simulink model "Cell_model_final4"  (R2023a)
settings: Solver=VariableStepAuto  StartTime=0.0  StopTime=T_e  FixedStep=0.005  RelTol=0.1
undefined symbols (not defined in the file or in its folder): C1_253, C1_263, C1_273, C1_283, C1_298, OCV_253, OCV_263, OCV_273, OCV_283, OCV_298, R0_253, R0_263, R0_273, R0_283, R0_298, R1_253, R1_263, R1_273, R1_283, R1_298
libraries: nesl_utility x8, fl_lib x7, dspstat3 x3, BatteryEstimators x1, deeplib x1, ee_lib x1, spspowerguiLib x1
settings Model: Creator=Lenovo  LastModifiedBy=Lenovo
settings DebuggingCC: AlgebraicLoopMsg=none

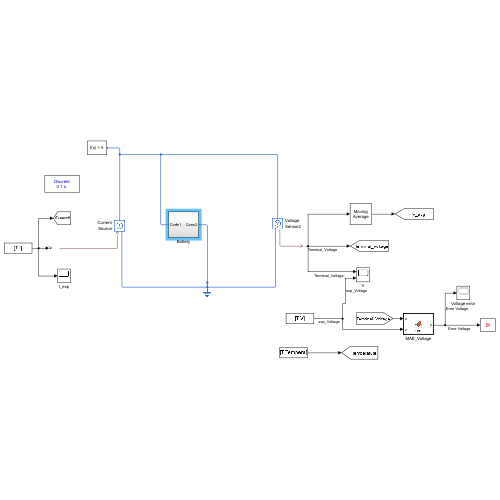
[thumbnail: Simulink's stored preview of the top-level diagram]
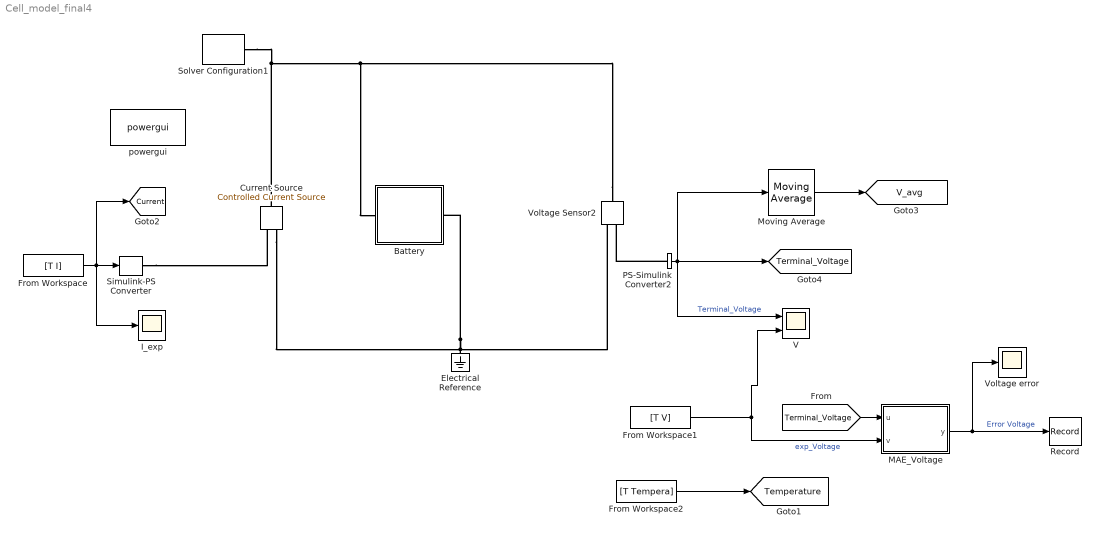
== system Cell_model_final4 ==
  Battery : Subsystem
  Current Source : fl_lib/Electrical/Electrical Sources/Controlled Current Source
  Electrical Reference : fl_lib/Electrical/Electrical Elements/Electrical Reference
  From Workspace : FromWorkspace  VariableName=[T I]
  From Workspace1 : FromWorkspace  VariableName=[T V]
  From Workspace2 : FromWorkspace  VariableName=[T Tempera]
  I_exp : Scope
  MAE_Voltage : MATLAB Function  TreatAsAtomicUnit=on
  Moving Average : dspstat3/Moving Average  Method=Sliding window  ForgettingFactorPort=off  SpecifyWindowLength=on  WindowLength=600  OverlapLength=599  AllowArbitraryInputLength=off  ForgettingFactor=0.9  SimulateUsing=Code generation
  PS-Simulink Converter2 : nesl_utility/PS-Simulink Converter  PhysicalDomain=network_engine_domain  SubClassName=ps_output  LeftPortType=input  RightPortType=output  PseudoPeriodic=off  Frequencies=[]  VectorFormat=1-D array  Unit=V  AffineConversion=off
  Record : Record  FileSettingsInternal="{\"entries\":[{\"content\":{\"excelSettings\":{\"content\":{},\"type\":\"Streamout.ExcelSettings\"}},\"type\":\"Streamout.FileSettingStorage\",\"uuid\":\"ccaf1daf-0eb7-4141-93b9-257bac153734\"}],\"packageUris\":[\"http://schema.mathworks.com/mf0/streamout_blocks/R2020a\"],\"version\":\"1.0\"}"  SignalsInternal="{\"entries\":[{\"content\":{\"signals\":[{\"content\":{\"blockPath\":[\"Cell_model_final4/Record\"],\"dimensions\":[1],\"domain\":\"Cell_model_final4/Record\",\"lineColor\":\"#a2142f\",\"plots\":[1],\"port\":1,\"sid\":[\"\"],\"signalID\":228,\"signalName\":\"Error Voltage\"},\"type\":\"RecordBlkView.Signal\",\"uuid\":\"8161d02f-5d6f-4f2d-b72f-e0f8d4715f56\"}]},\"type\":\"RecordBlkView.InputSignals\",\"uuid\":\"ac346876-ca78-426d-94f9-f8beec700152\"}],\"packageUris\":[\"http://schema.mathworks.com/mf0/streamout_blocks/R2020a\"],\"version\":\"1.0\"}"  VisualizationBindings="{\"sparklinesplugin\":{\"info\":[{\"bindingParametersList\":[],\"subplotID\":1}]}}"
  Simulink-PS Converter : nesl_utility/Simulink-PS Converter  PhysicalDomain=network_engine_domain  SubClassName=ps_input  LeftPortType=input  RightPortType=output  PseudoPeriodic=off  Frequencies=[]  NoiseDistribution=none  NoiseParameters=[]  Unit=A  AffineConversion=off  FilteringAndDerivatives=zero  SimscapeFilterOrder=1  InputFilterTimeConstant=.001  UdotUserProvided=0
  Solver Configuration1 : nesl_utility/Solver Configuration  PhysicalDomain=network_engine_domain  SubClassName=solver  LeftPortType=input  RightPortType=generic  Tones=[]  Harmonics=[]  SimulateNoise=off  Profile=off  UseLocalSampling=off  EnableSwitchedLinearOptims=on  FrequencyDomain=off  UseCCode=off  RelTol=0.001  AbsTol=0.001  MinStep=1e-09  ToWorkspace=off  RevertToSquareIcSolve=off  NumHomotopyIterations=100  PhasorMode=off  PhasorModeNumHarmonics=1  ConsistencySolver=NEWTON_XTOL_AFTER_FTOL  IndexReductionMethod=DerivativeReplacement  DoDC=off  ResidualTolerance=1e-09  ConsistencyTolSource=GLOBAL  ConsistencyAbsTol=0.001  ConsistencyRelTol=0.001  ConsistencyTolFactor=0.001  UseLocalSolver=off  LocalSolverChoice=NE_BACKWARD_EULER_ADVANCER  ResolveIndetEquations=on  FunctionEvalNumThread=1  LocalSolverSampleTime=0.001  DoFixedCost=off  MaxNonlinIter=3  MaxModeIter=2  ComputeImpulses=off  ImpulseIterations=2  LinearAlgebra=auto  LinearAlgebraNumThread=0  EquationFormulation=NE_TIME_EF  DelaysMemoryBudget=1024  AutomaticFiltering=on  FilteringTimeConstant=0.001  PartitionStorageMethod=AS_NEEDED  PartitionMemoryBudget=1024  PartitionMethod=ROBUST
  V : Scope  NumInputPorts=2
  Voltage Sensor2 : fl_lib/Electrical/Electrical Sensors/Voltage Sensor
  Voltage error : Scope
  powergui : spspowerguiLib/powergui  Priority=1  SimulationMode=Discrete  SampleTime=0.1  frequency=60  Iterations=50  frequencyindice=60  Pbase=100e6  ErrMax=1e-4  UnitsV=kV  UnitsW=MW  buscounter=0  FunctionMessages=off  echomessages=off  EnableUseOfTLC=off  CurrentSourceSwitches=off  DisableSnubberDevices=off  DisableRonSwitches=off  DisableVfSwitches=off  DisplayEquations=off  AutomaticDiscreteSolvers=off  SolverType=Tustin/Backward Euler (TBE)  Interpol=off  ExternalGateDelay=off  methode=off  Ts=100  x0status=blocks  SPID=on  SwTol=0  HookPort=off  NonlinearTolerance=1e-4  nMaxIteration=100  ContinueOnMaxIteration=off  RestoreLinks=warning  ResistiveCurrentMeasurement=off  Frange=[0:2:500]  Ylog=off  Xlog=on  ShowGrid=off  save=off  variable=ZData  structure=0  ZoomFFT=off  StartTime=0.0  cycles=1  DisplayStyle=1  fundamental=60  FreqAxis=off  MaxFrequency=1000  frequencyindicesteady=1  RmsSteady=1  display=off
  tag scope: Current=global, Temperature=global, Terminal_Voltage=global, V_avg=global
  wires:
  Moving Average/1 -> [V_avg]
  PS-Simulink Converter2/1 -> Moving Average/1, V/1, [Terminal_Voltage]  "Terminal_Voltage"
  From Workspace/1 -> I_exp/1, [Current], Simulink-PS Converter/1
  MAE_Voltage/1(y) -> Voltage error/1, Record/1  "Error Voltage"
  From Workspace1/1 -> V/2, MAE_Voltage/2(v)  "exp_Voltage"
  From Workspace2/1 -> [Temperature]
  [Terminal_Voltage] -> MAE_Voltage/1(u)
  connections:
  Voltage Sensor2/RConn2 -- Current Source/RConn2 -- Electrical Reference/LConn1 -- Battery/RConn1
  Voltage Sensor2/LConn1 -- Solver Configuration1/RConn1 -- Current Source/LConn1 -- Battery/LConn1
  Simulink-PS Converter/RConn1 -- Current Source/RConn1
  PS-Simulink Converter2/LConn1 -- Voltage Sensor2/RConn1

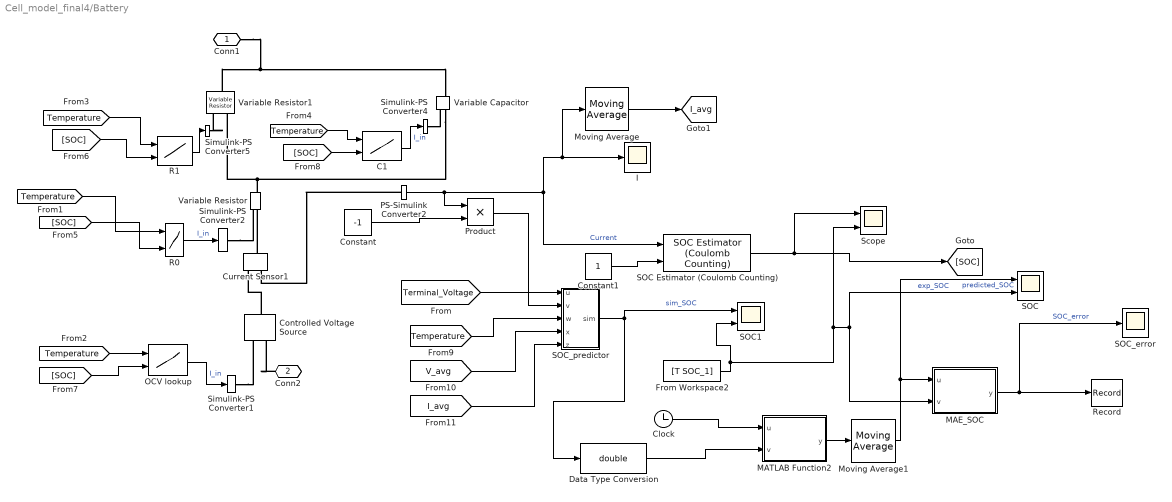
== system Cell_model_final4/Battery ==
  C1 : Lookup_n-D  BreakpointsForDimension1=[253;263;273;283;298]  BreakpointsForDimension2=[0;0.1;0.2;0.3;0.4;0.5;0.6;0.7;0.8;0.9;1]  Table=[C1_253;C1_263;C1_273;C1_283;C1_298]  InternalRulePriority=Speed  RndMeth=Simplest
      settings: InputPortMap=u0,u1
  Clock : Clock
  Constant : Constant  Value=-1
  Constant1 : Constant
  Controlled Voltage Source : fl_lib/Electrical/Electrical Sources/Controlled Voltage Source
  Current Sensor1 : fl_lib/Electrical/Electrical Sensors/Current Sensor
  Data Type Conversion : DataTypeConversion  OutDataTypeStr=double  SaturateOnIntegerOverflow=off  RndMeth=Floor
  From Workspace2 : FromWorkspace  VariableName=[T SOC_1]
  I : Scope
  MAE_SOC : MATLAB Function  TreatAsAtomicUnit=on
  MATLAB Function2 : MATLAB Function  TreatAsAtomicUnit=on
  Moving Average : dspstat3/Moving Average  Method=Sliding window  ForgettingFactorPort=off  SpecifyWindowLength=on  WindowLength=600  OverlapLength=599  AllowArbitraryInputLength=off  ForgettingFactor=0.9  SimulateUsing=Code generation
  Moving Average1 : dspstat3/Moving Average  Method=Sliding window  ForgettingFactorPort=off  SpecifyWindowLength=on  WindowLength=600  OverlapLength=599  AllowArbitraryInputLength=off  ForgettingFactor=0.9  SimulateUsing=Code generation
  OCV lookup : Lookup_n-D  BreakpointsForDimension1=[253;263;273;283;298]  BreakpointsForDimension2=[0;0.1;0.2;0.3;0.4;0.5;0.6;0.7;0.8;0.9;1]  Table=[OCV_253;OCV_263;OCV_273;OCV_283;OCV_298]  InternalRulePriority=Speed  RndMeth=Simplest
      settings: InputPortMap=u0,u1
  PS-Simulink Converter2 : nesl_utility/PS-Simulink Converter  PhysicalDomain=network_engine_domain  SubClassName=ps_output  LeftPortType=input  RightPortType=output  PseudoPeriodic=off  Frequencies=[]  VectorFormat=1-D array  Unit=A  AffineConversion=off
  Product : Product
  R0 : Lookup_n-D  BreakpointsForDimension1=[253;263;273;283;298]  BreakpointsForDimension2=[0;0.1;0.2;0.3;0.4;0.5;0.6;0.7;0.8;0.9;1]  Table=[R0_253;R0_263;R0_273;R0_283;R0_298]  InternalRulePriority=Speed  RndMeth=Simplest
      settings: InputPortMap=u0,u1
  R1 : Lookup_n-D  BreakpointsForDimension1=[253;263;273;283;298]  BreakpointsForDimension2=[0;0.1;0.2;0.3;0.4;0.5;0.6;0.7;0.8;0.9;1]  Table=[R1_253;R1_263;R1_273;R1_283;R1_298]  InternalRulePriority=Speed  RndMeth=Simplest
      settings: InputPortMap=u0,u1
  Record : Record  FileSettingsInternal="{\"entries\":[{\"content\":{\"excelSettings\":{\"content\":{},\"type\":\"Streamout.ExcelSettings\"}},\"type\":\"Streamout.FileSettingStorage\",\"uuid\":\"4492bafd-2dc4-4cd0-8cf0-f61798b460af\"}],\"packageUris\":[\"http://schema.mathworks.com/mf0/streamout_blocks/R2020a\"],\"version\":\"1.0\"}"  SignalsInternal="{\"entries\":[{\"content\":{\"signals\":[{\"content\":{\"blockPath\":[\"Cell_model_final4/Battery/Record\"],\"dimensions\":[1],\"domain\":\"Cell_model_final4/Battery/Record\",\"lineColor\":\"#139fff\",\"plots\":[1],\"port\":1,\"sid\":[\"\"],\"signalID\":232,\"signalName\":\"SOC_error\"},\"type\":\"RecordBlkView.Signal\",\"uuid\":\"cd1a7c72-596a-4650-bde3-9b31eae5e432\"}]},\"type\":\"RecordBlkView.InputSignals\",\"uuid\":\"78da0c69-a6e8-451d-b8ce-dbeaf7244afc\"}],\"packageUris\":[\"http://schema.mathworks.com/mf0/streamout_blocks/R2020a\"],\"version\":\"1.0\"}"  VisualizationBindings="{\"sparklinesplugin\":{\"info\":[{\"bindingParametersList\":[],\"subplotID\":1}]}}"
  SOC : Scope  NumInputPorts=2
  SOC Estimator (Coulomb Counting) : BatteryEstimators/SOC Estimator (Coulomb Counting)  AH=2.9  Ts=1
      settings: LibrarySourceBlock=|
      | batt_sl_lib/Estimators/SOC Estimator
      | (Coulomb Counting)
  SOC1 : Scope  NumInputPorts=2
  SOC_error : Scope
  SOC_predictor : Subsystem
  Scope : Scope  NumInputPorts=2
  Simulink-PS Converter1 : nesl_utility/Simulink-PS Converter  PhysicalDomain=network_engine_domain  SubClassName=ps_input  LeftPortType=input  RightPortType=output  PseudoPeriodic=off  Frequencies=[]  NoiseDistribution=none  NoiseParameters=[]  Unit=V  AffineConversion=off  FilteringAndDerivatives=zero  SimscapeFilterOrder=1  InputFilterTimeConstant=.001  UdotUserProvided=0
  Simulink-PS Converter2 : nesl_utility/Simulink-PS Converter  PhysicalDomain=network_engine_domain  SubClassName=ps_input  LeftPortType=input  RightPortType=output  PseudoPeriodic=off  Frequencies=[]  NoiseDistribution=none  NoiseParameters=[]  Unit=Ohm  AffineConversion=off  FilteringAndDerivatives=zero  SimscapeFilterOrder=1  InputFilterTimeConstant=.001  UdotUserProvided=0
  Simulink-PS Converter4 : nesl_utility/Simulink-PS Converter  PhysicalDomain=network_engine_domain  SubClassName=ps_input  LeftPortType=input  RightPortType=output  PseudoPeriodic=off  Frequencies=[]  NoiseDistribution=none  NoiseParameters=[]  Unit=F  AffineConversion=off  FilteringAndDerivatives=zero  SimscapeFilterOrder=1  InputFilterTimeConstant=.001  UdotUserProvided=0
  Simulink-PS Converter5 : nesl_utility/Simulink-PS Converter  PhysicalDomain=network_engine_domain  SubClassName=ps_input  LeftPortType=input  RightPortType=output  PseudoPeriodic=off  Frequencies=[]  NoiseDistribution=none  NoiseParameters=[]  Unit=Ohm  AffineConversion=on  FilteringAndDerivatives=provide  SimscapeFilterOrder=1  InputFilterTimeConstant=0.001  UdotUserProvided=0
  Variable Capacitor : ee_lib/Passive/Variable Capacitor  prm=2  Cmin=1e-9 F  r=1e-6 Ohm  v0=0 V  q0=0 C
      settings: InternalSimscapePortConfiguration="{\"Bottom\":[],\"Left\":[{\"id\":\"C\",\"label\":\"C\",\"type\":\"input\"},{\"id\":\"p\",\"label\":\"+\",\"type\":\"foundation.electrical.electrical\"}],\"Right\":[{\"id\":\"n\",\"label\":\"-\",\"type\":\"foundation.electrical.electrical\"}],\"Top\":[]}"
  Variable Resistor : fl_lib/Electrical/Electrical Elements/Variable Resistor  Rmin=0 Ohm  i_specify=off  i_priority=None  i=0 A  i_nominal_specify=off  i_nominal_unit=A  i_nominal_value=1  v_specify=off  v_priority=None  v=0 V  v_nominal_specify=off  v_nominal_unit=V  v_nominal_value=1
  Variable Resistor1 : fl_lib/Electrical/Electrical Elements/Variable Resistor  Rmin=0 Ohm  i_specify=off  i_priority=None  i=0 A  i_nominal_specify=off  i_nominal_unit=A  i_nominal_value=1  v_specify=off  v_priority=None  v=0 V  v_nominal_specify=off  v_nominal_unit=V  v_nominal_value=1
  Conn1 : PMIOPort  Side=Left
  Conn2 : PMIOPort  Port=2  Side=Right
  tag scope: I_avg=global
  wires:
  [Temperature] -> R0/1
  [SOC] -> R0/2
  [SOC] -> R1/2
  [Temperature] -> R1/1
  R1/1 -> Simulink-PS Converter5/1
  C1/1 -> Simulink-PS Converter4/1  "I_in"
  [Temperature] -> C1/1
  [SOC] -> C1/2
  PS-Simulink Converter2/1 -> Moving Average/1, I/1, SOC Estimator (Coulomb Counting)/1, Product/1  "Current"
  [Temperature] -> SOC_predictor/3(w)
  From Workspace2/1 -> SOC1/2, Scope/2, MAE_SOC/2(v), SOC/2  "exp_SOC"
  [Terminal_Voltage] -> SOC_predictor/1(u)
  [SOC] -> OCV lookup/2
  [Temperature] -> OCV lookup/1
  OCV lookup/1 -> Simulink-PS Converter1/1  "I_in"
  R0/1 -> Simulink-PS Converter2/1  "I_in"
  MAE_SOC/1(y) -> SOC_error/1, Record/1  "SOC_error"
  [V_avg] -> SOC_predictor/4(x)
  Moving Average/1 -> [I_avg]
  [I_avg] -> SOC_predictor/5(z)
  Constant/1 -> Product/2
  Product/1 -> SOC_predictor/2(v)
  Clock/1 -> MATLAB Function2/1(u)
  SOC_predictor/1(sim) -> SOC1/1, Data Type Conversion/1  "sim_SOC"
  Data Type Conversion/1 -> MATLAB Function2/2(v)
  SOC Estimator (Coulomb Counting)/1 -> Scope/1, [SOC]
  MATLAB Function2/1(y) -> Moving Average1/1
  Constant1/1 -> SOC Estimator (Coulomb Counting)/2
  Moving Average1/1 -> MAE_SOC/1(u), SOC/1  "predicted_SOC"
  connections:
  Simulink-PS Converter4/RConn1 -- Variable Capacitor/LConn1
  Simulink-PS Converter5/RConn1 -- Variable Resistor1/LConn1
  Variable Resistor/RConn1 -- Variable Resistor1/LConn2 -- Variable Capacitor/LConn2
  Simulink-PS Converter1/RConn1 -- Controlled Voltage Source/RConn1
  Variable Resistor1/RConn1 -- Conn1/RConn1 -- Variable Capacitor/RConn1
  Conn2/RConn1 -- Controlled Voltage Source/RConn2
  Simulink-PS Converter2/RConn1 -- Variable Resistor/LConn1
  Controlled Voltage Source/LConn1 -- Current Sensor1/RConn2
  Current Sensor1/LConn1 -- Variable Resistor/LConn2
  PS-Simulink Converter2/LConn1 -- Current Sensor1/RConn1

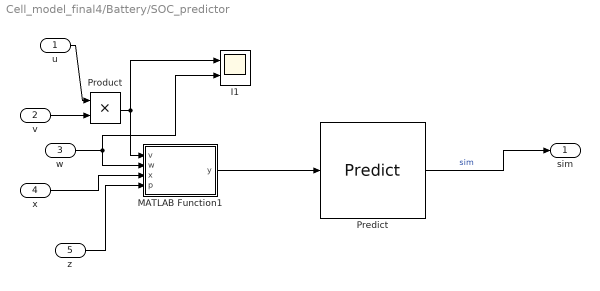
== system Cell_model_final4/Battery/SOC_predictor ==
  u : Inport
  v : Inport  Port=2
  w : Inport  Port=3
  x : Inport  Port=4
  z : Inport  Port=5
  I1 : Scope  NumInputPorts=2
  MATLAB Function1 : MATLAB Function  TreatAsAtomicUnit=on
  Predict : deeplib/Predict  Network=Network from MAT-file  NetworkFunction=squeezenet  NetworkFilePath=D:\Projects\Final_Year_Project\simulation\our_simulation\nets9.mat  MiniBatchSize=1  InputDataFormats={'',''}  Predictions=on  Activations={}  ForceInterpretedSim=off  EnableDLNetwork=on
  Product : Product
  sim : Outport
  wires:
  u/1 -> Product/1
  v/1 -> Product/2
  w/1 -> MATLAB Function1/2(w), I1/2
  MATLAB Function1/1(y) -> Predict/1
  x/1 -> MATLAB Function1/3(x)
  z/1 -> MATLAB Function1/4(p)
  Predict/1 -> sim/1  "sim"
  Product/1 -> MATLAB Function1/1(v), I1/1

== matlab function Cell_model_final4/Battery/MAE_SOC ==
  data: u input; y output; v input
function y = fcn(u,v)


y =abs(u-v);

== matlab function Cell_model_final4/Battery/SOC_predictor/MATLAB Function1 ==
  data: v input; y output; w input; x input; p input
function y = fcn(v,w,x,p)
  
    all=[v;w;x;p];

y = all;

== matlab function Cell_model_final4/MAE_Voltage ==
  data: u input; y output; v input
function y = fcn(u,v)


y =abs(u-v);

== matlab function Cell_model_final4/Battery/MATLAB Function2 ==
  data: u input; y output; v input
function y = fcn(u,v)
  
   if u<10
       y=1;
   else
       y = v;
   end
